simulink model "multi_rotor_sim"  (R2023b)
settings: Solver=ode4  StartTime=0.0  StopTime=inf  FixedStep=ST  RelTol=1e-3
values from neighbouring files (symbols this model uses):
  a0 = 0    [parameters.m]
  ASLOPE = 5.9    [parameters.m]
  Ax = 0.023    [parameters.m]
  Ay = 0.023    [parameters.m]
  Az = 0.106    [parameters.m]
  BLADES = 2    [parameters.m]
  BLCG = 0    [parameters.m]
  BLCP = 0    [parameters.m]
  BLH1 = b*sind(30)    [parameters.m]
  BLH2 = b    (= 0.275)    [parameters.m]
  BLH3 = b*sind(30)    [parameters.m]
  BLH4 = -b*sind(30)    [parameters.m]
  BLH5 = -b    (= -0.275)    [parameters.m]
  BLH6 = -b*sind(30)    [parameters.m]
  chi1 = 1    [parameters.m]
  chi2 = -1    [parameters.m]
  chi3 = 1    [parameters.m]
  chi4 = -1    [parameters.m]
  chi5 = 1    [parameters.m]
  chi6 = -1    [parameters.m]
  CHORD = 17.55e-3    (= 0.01755)    [parameters.m]
  CHORD75 = 21e-3    (= 0.021)    [parameters.m]
  dyn_viscosity = 17.89e-6    (= 1.789e-05)    [parameters.m]
  g0 = 9.80665    [parameters.m]
  href = 0    [parameters.m]
  k_ind = 1.35    [parameters.m]
  k_Omega = 14.92    [parameters.m]
  latref = 44.200626    [parameters.m]
  lonref = 12.063822    [parameters.m]
  m = 2.15    [parameters.m]
  MC_ATT_PITCH = 45*pi/180    (= 0.785398163397)    [parameters.m]
  MC_ATT_ROLL = 45*pi/180    (= 0.785398163397)    [parameters.m]
  MC_PITCH_P = 2    [parameters.m]
  MC_PITCHRATE_D = 0    [parameters.m]
  MC_PITCHRATE_I = 0.05    [parameters.m]
  MC_PITCHRATE_P = 0.09*3    (= 0.27)    [parameters.m]
  MC_RATE_PITCH = 500*pi/180    (= 8.72664625997)    [parameters.m]
  MC_RATE_ROLL = 500*pi/180    (= 8.72664625997)    [parameters.m]
  MC_RATE_YAW = 300*pi/180    (= 5.23598775598)    [parameters.m]
  MC_ROLL_P = 2    [parameters.m]
  MC_ROLLRATE_D = 0    [parameters.m]
  MC_ROLLRATE_I = 0.05    [parameters.m]
  MC_ROLLRATE_P = 0.09*3    (= 0.27)    [parameters.m]
  MC_VEL_FWD = 15    [parameters.m]
  MC_VEL_FWD_OPT = 0.5    [parameters.m]
  MC_VEL_LAT = 15    [parameters.m]
  MC_VEL_LAT_OPT = 0.5    [parameters.m]
  MC_VEL_VERT = 15    [parameters.m]
  MC_YAW_P = 0.55    [parameters.m]
  MC_YAWRATE_D = 0.05    [parameters.m]
  MC_YAWRATE_I = 0.02    [parameters.m]
  MC_YAWRATE_P = 0.15*3    (= 0.45)    [parameters.m]
  MPC_XY_VEL_D_ACC = 0.6    [parameters.m]
  MPC_XY_VEL_I_ACC = 0.8    [parameters.m]
  MPC_XY_VEL_P_ACC = 1.7    [parameters.m]
  MPC_Z_VEL_D_ACC = 0    [parameters.m]
  MPC_Z_VEL_I_ACC = 2    [parameters.m]
  MPC_Z_VEL_P_ACC = 4    [parameters.m]
  n = 0.6359    [parameters.m]
  p00 = 7.145e-2    (= 0.07145)    [parameters.m]
  p01 = 0.4377    [parameters.m]
  p02 = -10.13    [parameters.m]
  p10 = 1.259e-3    (= 0.001259)    [parameters.m]
  p11 = 1.284e-3    (= 0.001284)    [parameters.m]
  p20 = -7.513e-7    (= -7.513e-07)    [parameters.m]
  PWM_hover = (PWM_idle+PWM_max)/2    (= 1550)    [parameters.m]
  PWM_idle = 1100    [parameters.m]
  PWM_max = 2000    [parameters.m]
  ROTOR = 4*0.0254    (= 0.1016)    [parameters.m]
  ST = 0.01    [parameters.m]
  STACG = 0    [parameters.m]
  STACP = 0    [parameters.m]
  STAH1 = -b*cosd(30)    [parameters.m]
  STAH2 = 0    [parameters.m]
  STAH3 = b*cosd(30)    [parameters.m]
  STAH4 = b*cosd(30)    [parameters.m]
  STAH5 = 0    [parameters.m]
  STAH6 = -b*cosd(30)    [parameters.m]
  TERMINAL_SPEED = 0.5    [parameters.m]
  Theta0 = 45*pi/180    (= 0.785398163397)    [parameters.m]
  THETT = -38.0973*pi/180    (= -0.66492332112)    [parameters.m]
  wind_rate = [ 0 0 0 ]'    [parameters.m]
  wind_velocity_e = [ 0 0 0 ]'    [parameters.m]
  WLCG = -0.02    [parameters.m]
  WLCP = -0.08    [parameters.m]
  WLH1 = 32e-3    (= 0.032)    [parameters.m]
  WLH2 = 32e-3    (= 0.032)    [parameters.m]
  WLH3 = 32e-3    (= 0.032)    [parameters.m]
  WLH4 = 32e-3    (= 0.032)    [parameters.m]
  WLH5 = 32e-3    (= 0.032)    [parameters.m]
  WLH6 = 32e-3    (= 0.032)    [parameters.m]
undefined symbols (not defined in the file or in its folder): Earth, WGS84, X, Y, Z
libraries: sm_lib x258, slpidlib x36, nesl_utility x15, sharedtransform x13, aerolibutil x4, aerolibanimutils x3, sharedutil x2, sim3dlib x1, uavsim3dlib x1, shared6dof x1, aerolibtransform2 x1, aerolibatmos2 x1
(part 10 of 11)

== system multi_rotor_sim/3D_visualization/SIMECHANICS 3D SCENE/SimMechanics/MotorD/DCBL_Assembly_CounterClockwise_4_Top_1_RIGID/Assem4DCBL_Assembly_CounterClockwise_4_Top_1_RIGID ==
  Mieng_chan_canh_quat_1_RIGID : Subsystem
  ReferenceFrame : sm_lib/Frames and Transforms/Reference Frame
  Tang_tren_DCBL_1_RIGID : Subsystem
  Transform : sm_lib/Frames and Transforms/Rigid Transform  TranslationMethod=None  TranslationStandardOffset=0  TranslationStandardOffsetUnits=m  TranslationStandardAxis=+Z  TranslationCartesianOffset=[0 0 0]  TranslationCartesianOffsetUnits=m  TranslationROffset=0  TranslationROffsetUnits=m  TranslationZOffset=0  TranslationZOffsetUnits=m  TranslationThetaOffset=0  TranslationThetaOffsetUnits=deg  RotationMethod=None  RotationAngleUnits=deg  RotationStandardAxis=+Z  RotationAngle=0  RotationArbitraryAxis=[0 0 1]  FollAlignAxisA=+X  BaseAlignAxisA=+Y  FollAlignAxisB=+Y  BaseAlignAxisB=+Z  RotationSequenceAxes=FollowerAxes  RotationSequence=XYX  RotationSequenceAngles=[0 0 0]  RotationSequenceAnglesUnits=deg  RotationMatrix=[1 0 0; 0 1 0; 0 0 1]  Quaternion=[1 0 0 0]
  Transform1 : sm_lib/Frames and Transforms/Rigid Transform  TranslationMethod=Cartesian  TranslationStandardOffset=0  TranslationStandardOffsetUnits=mm  TranslationStandardAxis=+Z  TranslationCartesianOffset=[0 12.200000000000017 0]  TranslationCartesianOffsetUnits=mm  TranslationROffset=0  TranslationROffsetUnits=m  TranslationZOffset=0  TranslationZOffsetUnits=m  TranslationThetaOffset=0  TranslationThetaOffsetUnits=deg  RotationMethod=ArbitraryAxis  RotationAngleUnits=rad  RotationStandardAxis=+Z  RotationAngle=3.1415926535897931  RotationArbitraryAxis=[0 1 0]  FollAlignAxisA=+X  BaseAlignAxisA=+Y  FollAlignAxisB=+Y  BaseAlignAxisB=+Z  RotationSequenceAxes=FollowerAxes  RotationSequence=XYX  RotationSequenceAngles=[0 0 0]  RotationSequenceAnglesUnits=deg  RotationMatrix=[1 0 0; 0 1 0; 0 0 1]  Quaternion=[1 0 0 0]
  Transform2 : sm_lib/Frames and Transforms/Rigid Transform  TranslationMethod=Cartesian  TranslationStandardOffset=0  TranslationStandardOffsetUnits=mm  TranslationStandardAxis=+Z  TranslationCartesianOffset=[5.0000000000000044 5.5000000000000053 3.8000000000000118]  TranslationCartesianOffsetUnits=mm  TranslationROffset=0  TranslationROffsetUnits=m  TranslationZOffset=0  TranslationZOffsetUnits=m  TranslationThetaOffset=0  TranslationThetaOffsetUnits=deg  RotationMethod=ArbitraryAxis  RotationAngleUnits=rad  RotationStandardAxis=+Z  RotationAngle=3.1415926535897931  RotationArbitraryAxis=[0 1 0]  FollAlignAxisA=+X  BaseAlignAxisA=+Y  FollAlignAxisB=+Y  BaseAlignAxisB=+Z  RotationSequenceAxes=FollowerAxes  RotationSequence=XYX  RotationSequenceAngles=[0 0 0]  RotationSequenceAnglesUnits=deg  RotationMatrix=[1 0 0; 0 1 0; 0 0 1]  Quaternion=[1 0 0 0]
  Transform3 : sm_lib/Frames and Transforms/Rigid Transform  TranslationMethod=Cartesian  TranslationStandardOffset=0  TranslationStandardOffsetUnits=mm  TranslationStandardAxis=+Z  TranslationCartesianOffset=[0 16.899999999999999 0]  TranslationCartesianOffsetUnits=mm  TranslationROffset=0  TranslationROffsetUnits=m  TranslationZOffset=0  TranslationZOffsetUnits=m  TranslationThetaOffset=0  TranslationThetaOffsetUnits=deg  RotationMethod=ArbitraryAxis  RotationAngleUnits=rad  RotationStandardAxis=+Z  RotationAngle=2.0943951023931953  RotationArbitraryAxis=[-0.57735026918962584 0.57735026918962584 0.57735026918962584]  FollAlignAxisA=+X  BaseAlignAxisA=+Y  FollAlignAxisB=+Y  BaseAlignAxisB=+Z  RotationSequenceAxes=FollowerAxes  RotationSequence=XYX  RotationSequenceAngles=[0 0 0]  RotationSequenceAnglesUnits=deg  RotationMatrix=[1 0 0; 0 1 0; 0 0 1]  Quaternion=[1 0 0 0]
  Transform4 : sm_lib/Frames and Transforms/Rigid Transform  TranslationMethod=Cartesian  TranslationStandardOffset=0  TranslationStandardOffsetUnits=mm  TranslationStandardAxis=+Z  TranslationCartesianOffset=[0 30.500000000000014 0]  TranslationCartesianOffsetUnits=mm  TranslationROffset=0  TranslationROffsetUnits=m  TranslationZOffset=0  TranslationZOffsetUnits=m  TranslationThetaOffset=0  TranslationThetaOffsetUnits=deg  RotationMethod=ArbitraryAxis  RotationAngleUnits=rad  RotationStandardAxis=+Z  RotationAngle=2.994911156014171  RotationArbitraryAxis=[0 1 0]  FollAlignAxisA=+X  BaseAlignAxisA=+Y  FollAlignAxisB=+Y  BaseAlignAxisB=+Z  RotationSequenceAxes=FollowerAxes  RotationSequence=XYX  RotationSequenceAngles=[0 0 0]  RotationSequenceAnglesUnits=deg  RotationMatrix=[1 0 0; 0 1 0; 0 0 1]  Quaternion=[1 0 0 0]
  hex_nut_style_1_gradeab_iso_1_RIGID : Subsystem
  x10x4_7_counterclockwise_propeller_1_RIGID : Subsystem
  F : PMIOPort  Side=Left
  connections:
  Tang_tren_DCBL_1_RIGID/LConn1 -- Transform/RConn1
  Mieng_chan_canh_quat_1_RIGID/LConn1 -- Transform1/RConn1
  Transform2/RConn1 -- x10x4_7_counterclockwise_propeller_1_RIGID/LConn1
  Transform3/RConn1 -- hex_nut_style_1_gradeab_iso_1_RIGID/LConn1
  Transform/LConn1 -- Transform1/LConn1 -- Transform4/RConn1 -- ReferenceFrame/RConn1 -- Transform2/LConn1 -- Transform3/LConn1
  Transform4/LConn1 -- F/RConn1

== system multi_rotor_sim/3D_visualization/SIMECHANICS 3D SCENE/SimMechanics/Assembly_Quadrotor_NProp_1_RIGID/Assembly_Quadrotor_NoProp_1_RIGID/DCBL_Assembly_Clockwise_1_Bottom_1_RIGID/De_DCBL_1_RIGID ==
  ReferenceFrame : sm_lib/Frames and Transforms/Reference Frame
  Solid : sm_lib/Body Elements/File Solid  ExtGeomFileName=De_DCBL_Default_sldprt.STL  UnitType=Custom  ExtGeomFileUnits=mm  StepReaderType=HEX  ExportConvexHullGeometry=off  InertiaType=Custom  Mass=0.0094405067370886605  MassUnits=kg  CenterOfMass=[0 8.551755407943574 0]  CenterOfMassUnits=mm  MomentsOfInertia=[0.9581719720589793 0.57744869492610285 0.95817197205897908]  MomentsOfInertiaUnits=kg*mm^2  ProductsOfInertia=[0 -0.0012524646336928653 0]  ProductsOfInertiaUnits=kg*mm^2  BasedOnType=Density  Density=1000  DensityUnits=kg/(m^3)  DoExposeReferenceFrame=on  SerializedFrames=<Frames/>  GraphicType=FromGeometry  MarkerShape=Sphere  MarkerSize=10  MarkerSizeUnits=m  GraphicVisPropType=SimpleVisualProperties  GraphicDiffuseColor=[0.2 0.2 0.2]  GraphicSpecularColor=[0.5 0.5 0.5 1.0]  GraphicAmbientColor=[0.15 0.15 0.15 1.0]  GraphicEmissiveColor=[0.0 0.0 0.0 1.0]  GraphicShininess=75  GraphicOpacity=1
  F : PMIOPort  Side=Left
  connections:
  Solid/RConn1 -- ReferenceFrame/RConn1 -- F/RConn1

== system multi_rotor_sim/3D_visualization/SIMECHANICS 3D SCENE/SimMechanics/Assembly_Quadrotor_NProp_1_RIGID/Assembly_Quadrotor_NoProp_1_RIGID/DCBL_Assembly_Clockwise_3_Bottom_1_RIGID/De_DCBL_1_RIGID ==
  ReferenceFrame : sm_lib/Frames and Transforms/Reference Frame
  Solid : sm_lib/Body Elements/File Solid  ExtGeomFileName=De_DCBL_Default_sldprt.STL  UnitType=Custom  ExtGeomFileUnits=mm  StepReaderType=HEX  ExportConvexHullGeometry=off  InertiaType=Custom  Mass=0.0094405067370886605  MassUnits=kg  CenterOfMass=[0 8.551755407943574 0]  CenterOfMassUnits=mm  MomentsOfInertia=[0.9581719720589793 0.57744869492610285 0.95817197205897908]  MomentsOfInertiaUnits=kg*mm^2  ProductsOfInertia=[0 -0.0012524646336928653 0]  ProductsOfInertiaUnits=kg*mm^2  BasedOnType=Density  Density=1000  DensityUnits=kg/(m^3)  DoExposeReferenceFrame=on  SerializedFrames=<Frames/>  GraphicType=FromGeometry  MarkerShape=Sphere  MarkerSize=10  MarkerSizeUnits=m  GraphicVisPropType=SimpleVisualProperties  GraphicDiffuseColor=[0.2 0.2 0.2]  GraphicSpecularColor=[0.5 0.5 0.5 1.0]  GraphicAmbientColor=[0.15 0.15 0.15 1.0]  GraphicEmissiveColor=[0.0 0.0 0.0 1.0]  GraphicShininess=75  GraphicOpacity=1
  F : PMIOPort  Side=Left
  connections:
  Solid/RConn1 -- ReferenceFrame/RConn1 -- F/RConn1

== system multi_rotor_sim/3D_visualization/SIMECHANICS 3D SCENE/SimMechanics/Assembly_Quadrotor_NProp_1_RIGID/Assembly_Quadrotor_NoProp_1_RIGID/DCBL_Assembly_CounterClockwise_2_Bottom_1_RIGID/De_DCBL_1_RIGID ==
  ReferenceFrame : sm_lib/Frames and Transforms/Reference Frame
  Solid : sm_lib/Body Elements/File Solid  ExtGeomFileName=De_DCBL_Default_sldprt.STL  UnitType=Custom  ExtGeomFileUnits=mm  StepReaderType=HEX  ExportConvexHullGeometry=off  InertiaType=Custom  Mass=0.0094405067370886605  MassUnits=kg  CenterOfMass=[0 8.551755407943574 0]  CenterOfMassUnits=mm  MomentsOfInertia=[0.9581719720589793 0.57744869492610285 0.95817197205897908]  MomentsOfInertiaUnits=kg*mm^2  ProductsOfInertia=[0 -0.0012524646336928653 0]  ProductsOfInertiaUnits=kg*mm^2  BasedOnType=Density  Density=1000  DensityUnits=kg/(m^3)  DoExposeReferenceFrame=on  SerializedFrames=<Frames/>  GraphicType=FromGeometry  MarkerShape=Sphere  MarkerSize=10  MarkerSizeUnits=m  GraphicVisPropType=SimpleVisualProperties  GraphicDiffuseColor=[0.2 0.2 0.2]  GraphicSpecularColor=[0.5 0.5 0.5 1.0]  GraphicAmbientColor=[0.15 0.15 0.15 1.0]  GraphicEmissiveColor=[0.0 0.0 0.0 1.0]  GraphicShininess=75  GraphicOpacity=1
  F : PMIOPort  Side=Left
  connections:
  Solid/RConn1 -- ReferenceFrame/RConn1 -- F/RConn1

== system multi_rotor_sim/3D_visualization/SIMECHANICS 3D SCENE/SimMechanics/Assembly_Quadrotor_NProp_1_RIGID/Assembly_Quadrotor_NoProp_1_RIGID/DCBL_Assembly_CounterClockwise_4_Bottom_1_RIGID/De_DCBL_1_RIGID ==
  ReferenceFrame : sm_lib/Frames and Transforms/Reference Frame
  Solid : sm_lib/Body Elements/File Solid  ExtGeomFileName=De_DCBL_Default_sldprt.STL  UnitType=Custom  ExtGeomFileUnits=mm  StepReaderType=HEX  ExportConvexHullGeometry=off  InertiaType=Custom  Mass=0.0094405067370886605  MassUnits=kg  CenterOfMass=[0 8.551755407943574 0]  CenterOfMassUnits=mm  MomentsOfInertia=[0.9581719720589793 0.57744869492610285 0.95817197205897908]  MomentsOfInertiaUnits=kg*mm^2  ProductsOfInertia=[0 -0.0012524646336928653 0]  ProductsOfInertiaUnits=kg*mm^2  BasedOnType=Density  Density=1000  DensityUnits=kg/(m^3)  DoExposeReferenceFrame=on  SerializedFrames=<Frames/>  GraphicType=FromGeometry  MarkerShape=Sphere  MarkerSize=10  MarkerSizeUnits=m  GraphicVisPropType=SimpleVisualProperties  GraphicDiffuseColor=[0.2 0.2 0.2]  GraphicSpecularColor=[0.5 0.5 0.5 1.0]  GraphicAmbientColor=[0.15 0.15 0.15 1.0]  GraphicEmissiveColor=[0.0 0.0 0.0 1.0]  GraphicShininess=75  GraphicOpacity=1
  F : PMIOPort  Side=Left
  connections:
  Solid/RConn1 -- ReferenceFrame/RConn1 -- F/RConn1

== system multi_rotor_sim/3D_visualization/SIMECHANICS 3D SCENE/SimMechanics/MotorA/DCBL_Assembly_Clockwise_1_Top_1_RIGID/Assem1DCBL_Assembly_Clockwise_1_Top_1_RIGID/Mieng_chan_canh_quat_1_RIGID ==
  ReferenceFrame : sm_lib/Frames and Transforms/Reference Frame
  Solid : sm_lib/Body Elements/File Solid  ExtGeomFileName=Mieng_chan_canh_quat_Default_sldprt.STL  UnitType=Custom  ExtGeomFileUnits=mm  StepReaderType=HEX  ExportConvexHullGeometry=off  InertiaType=Custom  Mass=0.00066710164886432991  MassUnits=kg  CenterOfMass=[0 0.34100350204192958 0]  CenterOfMassUnits=mm  MomentsOfInertia=[0.0086037825507957657 0.016809111968954363 0.0086037825507957692]  MomentsOfInertiaUnits=kg*mm^2  ProductsOfInertia=[0 0 0]  ProductsOfInertiaUnits=kg*mm^2  BasedOnType=Density  Density=1000  DensityUnits=kg/(m^3)  DoExposeReferenceFrame=on  SerializedFrames=<Frames/>  GraphicType=FromGeometry  MarkerShape=Sphere  MarkerSize=10  MarkerSizeUnits=m  GraphicVisPropType=SimpleVisualProperties  GraphicDiffuseColor=[0.1 0.1 0.1]  GraphicSpecularColor=[0.5 0.5 0.5 1.0]  GraphicAmbientColor=[0.15 0.15 0.15 1.0]  GraphicEmissiveColor=[0.0 0.0 0.0 1.0]  GraphicShininess=75  GraphicOpacity=1
  F : PMIOPort  Side=Left
  connections:
  Solid/RConn1 -- ReferenceFrame/RConn1 -- F/RConn1

== system multi_rotor_sim/3D_visualization/SIMECHANICS 3D SCENE/SimMechanics/MotorA/DCBL_Assembly_Clockwise_1_Top_1_RIGID/Assem1DCBL_Assembly_Clockwise_1_Top_1_RIGID/Tang_tren_DCBL_1_RIGID ==
  ReferenceFrame : sm_lib/Frames and Transforms/Reference Frame
  Solid : sm_lib/Body Elements/File Solid  ExtGeomFileName=Tang_tren_DCBL_Default_sldprt.STL  UnitType=Custom  ExtGeomFileUnits=mm  StepReaderType=HEX  ExportConvexHullGeometry=off  InertiaType=Custom  Mass=0.0096533797201190392  MassUnits=kg  CenterOfMass=[0 -3.2502099324489322 0]  CenterOfMassUnits=mm  MomentsOfInertia=[1.2743807926810715 0.81038583319969226 1.2743807926810709]  MomentsOfInertiaUnits=kg*mm^2  ProductsOfInertia=[0 0 0]  ProductsOfInertiaUnits=kg*mm^2  BasedOnType=Density  Density=1000  DensityUnits=kg/(m^3)  DoExposeReferenceFrame=on  SerializedFrames=<Frames/>  GraphicType=FromGeometry  MarkerShape=Sphere  MarkerSize=10  MarkerSizeUnits=m  GraphicVisPropType=SimpleVisualProperties  GraphicDiffuseColor=[0.1 0.1 0.1]  GraphicSpecularColor=[0.5 0.5 0.5 1.0]  GraphicAmbientColor=[0.15 0.15 0.15 1.0]  GraphicEmissiveColor=[0.0 0.0 0.0 1.0]  GraphicShininess=75  GraphicOpacity=1
  F : PMIOPort  Side=Left
  connections:
  Solid/RConn1 -- ReferenceFrame/RConn1 -- F/RConn1

== system multi_rotor_sim/3D_visualization/SIMECHANICS 3D SCENE/SimMechanics/MotorA/DCBL_Assembly_Clockwise_1_Top_1_RIGID/Assem1DCBL_Assembly_Clockwise_1_Top_1_RIGID/hex_nut_style_1_gradeab_iso_1_RIGID ==
  ReferenceFrame : sm_lib/Frames and Transforms/Reference Frame
  Solid : sm_lib/Body Elements/File Solid  ExtGeomFileName=hex nut style 1 gradeab_iso_Hexagon Nut ISO - 4032 - M4 - D - N_sldprt.STL  UnitType=Custom  ExtGeomFileUnits=mm  StepReaderType=HEX  ExportConvexHullGeometry=off  InertiaType=Custom  Mass=0.00010662444846940384  MassUnits=kg  CenterOfMass=[0 1.3702747535691162e-06 -1.5985959803450969]  CenterOfMassUnits=mm  MomentsOfInertia=[0.00052487586358693401 0.00052487294180577238 0.00087302244809774987]  MomentsOfInertiaUnits=kg*mm^2  ProductsOfInertia=[0 0 0]  ProductsOfInertiaUnits=kg*mm^2  BasedOnType=Density  Density=1000  DensityUnits=kg/(m^3)  DoExposeReferenceFrame=on  SerializedFrames=<Frames/>  GraphicType=FromGeometry  MarkerShape=Sphere  MarkerSize=10  MarkerSizeUnits=m  GraphicVisPropType=SimpleVisualProperties  GraphicDiffuseColor=[0.77647058823529413 0.75686274509803919 0.73725490196078436]  GraphicSpecularColor=[0.5 0.5 0.5 1.0]  GraphicAmbientColor=[0.15 0.15 0.15 1.0]  GraphicEmissiveColor=[0.0 0.0 0.0 1.0]  GraphicShininess=75  GraphicOpacity=1
  F : PMIOPort  Side=Left
  connections:
  Solid/RConn1 -- ReferenceFrame/RConn1 -- F/RConn1

== system multi_rotor_sim/3D_visualization/SIMECHANICS 3D SCENE/SimMechanics/MotorA/DCBL_Assembly_Clockwise_1_Top_1_RIGID/Assem1DCBL_Assembly_Clockwise_1_Top_1_RIGID/x10x4_7_clockwise_propeller_1_RIGID ==
  ReferenceFrame : sm_lib/Frames and Transforms/Reference Frame
  Solid : sm_lib/Body Elements/File Solid  ExtGeomFileName=10x4.7-clockwise-propeller_Default_sldprt.STL  UnitType=Custom  ExtGeomFileUnits=mm  StepReaderType=HEX  ExportConvexHullGeometry=off  InertiaType=Custom  Mass=0.0085886554018527825  MassUnits=kg  CenterOfMass=[5.0000101361481475 5.1432840109255382 3.799999228152465]  CenterOfMassUnits=mm  MomentsOfInertia=[37.986675876119939 39.040615812058284 1.1185316341050053]  MomentsOfInertiaUnits=kg*mm^2  ProductsOfInertia=[-7.8946012766185134e-07 -5.513228057178063 2.3221541821947674e-07]  ProductsOfInertiaUnits=kg*mm^2  BasedOnType=Density  Density=1000  DensityUnits=kg/(m^3)  DoExposeReferenceFrame=on  SerializedFrames=<Frames/>  GraphicType=FromGeometry  MarkerShape=Sphere  MarkerSize=10  MarkerSizeUnits=m  GraphicVisPropType=SimpleVisualProperties  GraphicDiffuseColor=[0.75294117647058822 0.75294117647058822 0.75294117647058822]  GraphicSpecularColor=[0.5 0.5 0.5 1.0]  GraphicAmbientColor=[0.15 0.15 0.15 1.0]  GraphicEmissiveColor=[0.0 0.0 0.0 1.0]  GraphicShininess=75  GraphicOpacity=1
  F : PMIOPort  Side=Left
  connections:
  Solid/RConn1 -- ReferenceFrame/RConn1 -- F/RConn1

== system multi_rotor_sim/3D_visualization/SIMECHANICS 3D SCENE/SimMechanics/MotorB/DCBL_Assembly_CounterClockwise_2_Top_1_RIGID/Assem2DCBL_Assembly_CounterClockwise_2_Top_1_RIGID/Mieng_chan_canh_quat_1_RIGID ==
  ReferenceFrame : sm_lib/Frames and Transforms/Reference Frame
  Solid : sm_lib/Body Elements/File Solid  ExtGeomFileName=Mieng_chan_canh_quat_Default_sldprt.STL  UnitType=Custom  ExtGeomFileUnits=mm  StepReaderType=HEX  ExportConvexHullGeometry=off  InertiaType=Custom  Mass=0.00066710164886432991  MassUnits=kg  CenterOfMass=[0 0.34100350204192958 0]  CenterOfMassUnits=mm  MomentsOfInertia=[0.0086037825507957657 0.016809111968954363 0.0086037825507957692]  MomentsOfInertiaUnits=kg*mm^2  ProductsOfInertia=[0 0 0]  ProductsOfInertiaUnits=kg*mm^2  BasedOnType=Density  Density=1000  DensityUnits=kg/(m^3)  DoExposeReferenceFrame=on  SerializedFrames=<Frames/>  GraphicType=FromGeometry  MarkerShape=Sphere  MarkerSize=10  MarkerSizeUnits=m  GraphicVisPropType=SimpleVisualProperties  GraphicDiffuseColor=[0.1 0.1 0.1]  GraphicSpecularColor=[0.5 0.5 0.5 1.0]  GraphicAmbientColor=[0.15 0.15 0.15 1.0]  GraphicEmissiveColor=[0.0 0.0 0.0 1.0]  GraphicShininess=75  GraphicOpacity=1
  F : PMIOPort  Side=Left
  connections:
  Solid/RConn1 -- ReferenceFrame/RConn1 -- F/RConn1

== system multi_rotor_sim/3D_visualization/SIMECHANICS 3D SCENE/SimMechanics/MotorB/DCBL_Assembly_CounterClockwise_2_Top_1_RIGID/Assem2DCBL_Assembly_CounterClockwise_2_Top_1_RIGID/Tang_tren_DCBL_1_RIGID ==
  ReferenceFrame : sm_lib/Frames and Transforms/Reference Frame
  Solid : sm_lib/Body Elements/File Solid  ExtGeomFileName=Tang_tren_DCBL_Default_sldprt.STL  UnitType=Custom  ExtGeomFileUnits=mm  StepReaderType=HEX  ExportConvexHullGeometry=off  InertiaType=Custom  Mass=0.0096533797201190392  MassUnits=kg  CenterOfMass=[0 -3.2502099324489322 0]  CenterOfMassUnits=mm  MomentsOfInertia=[1.2743807926810715 0.81038583319969226 1.2743807926810709]  MomentsOfInertiaUnits=kg*mm^2  ProductsOfInertia=[0 0 0]  ProductsOfInertiaUnits=kg*mm^2  BasedOnType=Density  Density=1000  DensityUnits=kg/(m^3)  DoExposeReferenceFrame=on  SerializedFrames=<Frames/>  GraphicType=FromGeometry  MarkerShape=Sphere  MarkerSize=10  MarkerSizeUnits=m  GraphicVisPropType=SimpleVisualProperties  GraphicDiffuseColor=[0.1 0.1 0.1]  GraphicSpecularColor=[0.5 0.5 0.5 1.0]  GraphicAmbientColor=[0.15 0.15 0.15 1.0]  GraphicEmissiveColor=[0.0 0.0 0.0 1.0]  GraphicShininess=75  GraphicOpacity=1
  F : PMIOPort  Side=Left
  connections:
  Solid/RConn1 -- ReferenceFrame/RConn1 -- F/RConn1

== system multi_rotor_sim/3D_visualization/SIMECHANICS 3D SCENE/SimMechanics/MotorB/DCBL_Assembly_CounterClockwise_2_Top_1_RIGID/Assem2DCBL_Assembly_CounterClockwise_2_Top_1_RIGID/hex_nut_style_1_gradeab_iso_1_RIGID ==
  ReferenceFrame : sm_lib/Frames and Transforms/Reference Frame
  Solid : sm_lib/Body Elements/File Solid  ExtGeomFileName=hex nut style 1 gradeab_iso_Hexagon Nut ISO - 4032 - M4 - D - N_sldprt.STL  UnitType=Custom  ExtGeomFileUnits=mm  StepReaderType=HEX  ExportConvexHullGeometry=off  InertiaType=Custom  Mass=0.00010662444846940384  MassUnits=kg  CenterOfMass=[0 1.3702747535691162e-06 -1.5985959803450969]  CenterOfMassUnits=mm  MomentsOfInertia=[0.00052487586358693401 0.00052487294180577238 0.00087302244809774987]  MomentsOfInertiaUnits=kg*mm^2  ProductsOfInertia=[0 0 0]  ProductsOfInertiaUnits=kg*mm^2  BasedOnType=Density  Density=1000  DensityUnits=kg/(m^3)  DoExposeReferenceFrame=on  SerializedFrames=<Frames/>  GraphicType=FromGeometry  MarkerShape=Sphere  MarkerSize=10  MarkerSizeUnits=m  GraphicVisPropType=SimpleVisualProperties  GraphicDiffuseColor=[0.77647058823529413 0.75686274509803919 0.73725490196078436]  GraphicSpecularColor=[0.5 0.5 0.5 1.0]  GraphicAmbientColor=[0.15 0.15 0.15 1.0]  GraphicEmissiveColor=[0.0 0.0 0.0 1.0]  GraphicShininess=75  GraphicOpacity=1
  F : PMIOPort  Side=Left
  connections:
  Solid/RConn1 -- ReferenceFrame/RConn1 -- F/RConn1

== system multi_rotor_sim/3D_visualization/SIMECHANICS 3D SCENE/SimMechanics/MotorB/DCBL_Assembly_CounterClockwise_2_Top_1_RIGID/Assem2DCBL_Assembly_CounterClockwise_2_Top_1_RIGID/x10x4_7_counterclockwise_propeller_1_RIGID ==
  ReferenceFrame : sm_lib/Frames and Transforms/Reference Frame
  Solid : sm_lib/Body Elements/File Solid  ExtGeomFileName=10x4.7-counterclockwise-propeller_Default_sldprt.STL  UnitType=Custom  ExtGeomFileUnits=mm  StepReaderType=HEX  ExportConvexHullGeometry=off  InertiaType=Custom  Mass=0.0086221636611543556  MassUnits=kg  CenterOfMass=[5.0000063702530122 5.136767030722547 3.7999863031218535]  CenterOfMassUnits=mm  MomentsOfInertia=[38.086408780943664 39.145966882895458 1.124519086575168]  MomentsOfInertiaUnits=kg*mm^2  ProductsOfInertia=[-1.7703894482553841e-07 5.5344154529569156 1.457353668708178e-07]  ProductsOfInertiaUnits=kg*mm^2  BasedOnType=Density  Density=1000  DensityUnits=kg/(m^3)  DoExposeReferenceFrame=on  SerializedFrames=<Frames/>  GraphicType=FromGeometry  MarkerShape=Sphere  MarkerSize=10  MarkerSizeUnits=m  GraphicVisPropType=SimpleVisualProperties  GraphicDiffuseColor=[0.75294117647058822 0.75294117647058822 0.75294117647058822]  GraphicSpecularColor=[0.5 0.5 0.5 1.0]  GraphicAmbientColor=[0.15 0.15 0.15 1.0]  GraphicEmissiveColor=[0.0 0.0 0.0 1.0]  GraphicShininess=75  GraphicOpacity=1
  F : PMIOPort  Side=Left
  connections:
  Solid/RConn1 -- ReferenceFrame/RConn1 -- F/RConn1

== system multi_rotor_sim/3D_visualization/SIMECHANICS 3D SCENE/SimMechanics/MotorC/DCBL_Assembly_Clockwise_3_Top_1_RIGID/Assem3DCBL_Assembly_Clockwise_3_Top_1_RIGID/Mieng_chan_canh_quat_1_RIGID ==
  ReferenceFrame : sm_lib/Frames and Transforms/Reference Frame
  Solid : sm_lib/Body Elements/File Solid  ExtGeomFileName=Mieng_chan_canh_quat_Default_sldprt.STL  UnitType=Custom  ExtGeomFileUnits=mm  StepReaderType=HEX  ExportConvexHullGeometry=off  InertiaType=Custom  Mass=0.00066710164886432991  MassUnits=kg  CenterOfMass=[0 0.34100350204192958 0]  CenterOfMassUnits=mm  MomentsOfInertia=[0.0086037825507957657 0.016809111968954363 0.0086037825507957692]  MomentsOfInertiaUnits=kg*mm^2  ProductsOfInertia=[0 0 0]  ProductsOfInertiaUnits=kg*mm^2  BasedOnType=Density  Density=1000  DensityUnits=kg/(m^3)  DoExposeReferenceFrame=on  SerializedFrames=<Frames/>  GraphicType=FromGeometry  MarkerShape=Sphere  MarkerSize=10  MarkerSizeUnits=m  GraphicVisPropType=SimpleVisualProperties  GraphicDiffuseColor=[0.1 0.1 0.1]  GraphicSpecularColor=[0.5 0.5 0.5 1.0]  GraphicAmbientColor=[0.15 0.15 0.15 1.0]  GraphicEmissiveColor=[0.0 0.0 0.0 1.0]  GraphicShininess=75  GraphicOpacity=1
  F : PMIOPort  Side=Left
  connections:
  Solid/RConn1 -- ReferenceFrame/RConn1 -- F/RConn1

== system multi_rotor_sim/3D_visualization/SIMECHANICS 3D SCENE/SimMechanics/MotorC/DCBL_Assembly_Clockwise_3_Top_1_RIGID/Assem3DCBL_Assembly_Clockwise_3_Top_1_RIGID/Tang_tren_DCBL_1_RIGID ==
  ReferenceFrame : sm_lib/Frames and Transforms/Reference Frame
  Solid : sm_lib/Body Elements/File Solid  ExtGeomFileName=Tang_tren_DCBL_Default_sldprt.STL  UnitType=Custom  ExtGeomFileUnits=mm  StepReaderType=HEX  ExportConvexHullGeometry=off  InertiaType=Custom  Mass=0.0096533797201190392  MassUnits=kg  CenterOfMass=[0 -3.2502099324489322 0]  CenterOfMassUnits=mm  MomentsOfInertia=[1.2743807926810715 0.81038583319969226 1.2743807926810709]  MomentsOfInertiaUnits=kg*mm^2  ProductsOfInertia=[0 0 0]  ProductsOfInertiaUnits=kg*mm^2  BasedOnType=Density  Density=1000  DensityUnits=kg/(m^3)  DoExposeReferenceFrame=on  SerializedFrames=<Frames/>  GraphicType=FromGeometry  MarkerShape=Sphere  MarkerSize=10  MarkerSizeUnits=m  GraphicVisPropType=SimpleVisualProperties  GraphicDiffuseColor=[0.1 0.1 0.1]  GraphicSpecularColor=[0.5 0.5 0.5 1.0]  GraphicAmbientColor=[0.15 0.15 0.15 1.0]  GraphicEmissiveColor=[0.0 0.0 0.0 1.0]  GraphicShininess=75  GraphicOpacity=1
  F : PMIOPort  Side=Left
  connections:
  Solid/RConn1 -- ReferenceFrame/RConn1 -- F/RConn1

== system multi_rotor_sim/3D_visualization/SIMECHANICS 3D SCENE/SimMechanics/MotorC/DCBL_Assembly_Clockwise_3_Top_1_RIGID/Assem3DCBL_Assembly_Clockwise_3_Top_1_RIGID/hex_nut_style_1_gradeab_iso_1_RIGID ==
  ReferenceFrame : sm_lib/Frames and Transforms/Reference Frame
  Solid : sm_lib/Body Elements/File Solid  ExtGeomFileName=hex nut style 1 gradeab_iso_Hexagon Nut ISO - 4032 - M4 - D - N_sldprt.STL  UnitType=Custom  ExtGeomFileUnits=mm  StepReaderType=HEX  ExportConvexHullGeometry=off  InertiaType=Custom  Mass=0.00010662444846940384  MassUnits=kg  CenterOfMass=[0 1.3702747535691162e-06 -1.5985959803450969]  CenterOfMassUnits=mm  MomentsOfInertia=[0.00052487586358693401 0.00052487294180577238 0.00087302244809774987]  MomentsOfInertiaUnits=kg*mm^2  ProductsOfInertia=[0 0 0]  ProductsOfInertiaUnits=kg*mm^2  BasedOnType=Density  Density=1000  DensityUnits=kg/(m^3)  DoExposeReferenceFrame=on  SerializedFrames=<Frames/>  GraphicType=FromGeometry  MarkerShape=Sphere  MarkerSize=10  MarkerSizeUnits=m  GraphicVisPropType=SimpleVisualProperties  GraphicDiffuseColor=[0.77647058823529413 0.75686274509803919 0.73725490196078436]  GraphicSpecularColor=[0.5 0.5 0.5 1.0]  GraphicAmbientColor=[0.15 0.15 0.15 1.0]  GraphicEmissiveColor=[0.0 0.0 0.0 1.0]  GraphicShininess=75  GraphicOpacity=1
  F : PMIOPort  Side=Left
  connections:
  Solid/RConn1 -- ReferenceFrame/RConn1 -- F/RConn1

== system multi_rotor_sim/3D_visualization/SIMECHANICS 3D SCENE/SimMechanics/MotorC/DCBL_Assembly_Clockwise_3_Top_1_RIGID/Assem3DCBL_Assembly_Clockwise_3_Top_1_RIGID/x10x4_7_clockwise_propeller_1_RIGID ==
  ReferenceFrame : sm_lib/Frames and Transforms/Reference Frame
  Solid : sm_lib/Body Elements/File Solid  ExtGeomFileName=10x4.7-clockwise-propeller_Default_sldprt.STL  UnitType=Custom  ExtGeomFileUnits=mm  StepReaderType=HEX  ExportConvexHullGeometry=off  InertiaType=Custom  Mass=0.0085886554018527825  MassUnits=kg  CenterOfMass=[5.0000101361481475 5.1432840109255382 3.799999228152465]  CenterOfMassUnits=mm  MomentsOfInertia=[37.986675876119939 39.040615812058284 1.1185316341050053]  MomentsOfInertiaUnits=kg*mm^2  ProductsOfInertia=[-7.8946012766185134e-07 -5.513228057178063 2.3221541821947674e-07]  ProductsOfInertiaUnits=kg*mm^2  BasedOnType=Density  Density=1000  DensityUnits=kg/(m^3)  DoExposeReferenceFrame=on  SerializedFrames=<Frames/>  GraphicType=FromGeometry  MarkerShape=Sphere  MarkerSize=10  MarkerSizeUnits=m  GraphicVisPropType=SimpleVisualProperties  GraphicDiffuseColor=[0.75294117647058822 0.75294117647058822 0.75294117647058822]  GraphicSpecularColor=[0.5 0.5 0.5 1.0]  GraphicAmbientColor=[0.15 0.15 0.15 1.0]  GraphicEmissiveColor=[0.0 0.0 0.0 1.0]  GraphicShininess=75  GraphicOpacity=1
  F : PMIOPort  Side=Left
  connections:
  Solid/RConn1 -- ReferenceFrame/RConn1 -- F/RConn1

== system multi_rotor_sim/3D_visualization/SIMECHANICS 3D SCENE/SimMechanics/MotorD/DCBL_Assembly_CounterClockwise_4_Top_1_RIGID/Assem4DCBL_Assembly_CounterClockwise_4_Top_1_RIGID/Mieng_chan_canh_quat_1_RIGID ==
  ReferenceFrame : sm_lib/Frames and Transforms/Reference Frame
  Solid : sm_lib/Body Elements/File Solid  ExtGeomFileName=Mieng_chan_canh_quat_Default_sldprt.STL  UnitType=Custom  ExtGeomFileUnits=mm  StepReaderType=HEX  ExportConvexHullGeometry=off  InertiaType=Custom  Mass=0.00066710164886432991  MassUnits=kg  CenterOfMass=[0 0.34100350204192958 0]  CenterOfMassUnits=mm  MomentsOfInertia=[0.0086037825507957657 0.016809111968954363 0.0086037825507957692]  MomentsOfInertiaUnits=kg*mm^2  ProductsOfInertia=[0 0 0]  ProductsOfInertiaUnits=kg*mm^2  BasedOnType=Density  Density=1000  DensityUnits=kg/(m^3)  DoExposeReferenceFrame=on  SerializedFrames=<Frames/>  GraphicType=FromGeometry  MarkerShape=Sphere  MarkerSize=10  MarkerSizeUnits=m  GraphicVisPropType=SimpleVisualProperties  GraphicDiffuseColor=[0.1 0.1 0.1]  GraphicSpecularColor=[0.5 0.5 0.5 1.0]  GraphicAmbientColor=[0.15 0.15 0.15 1.0]  GraphicEmissiveColor=[0.0 0.0 0.0 1.0]  GraphicShininess=75  GraphicOpacity=1
  F : PMIOPort  Side=Left
  connections:
  Solid/RConn1 -- ReferenceFrame/RConn1 -- F/RConn1

== system multi_rotor_sim/3D_visualization/SIMECHANICS 3D SCENE/SimMechanics/MotorD/DCBL_Assembly_CounterClockwise_4_Top_1_RIGID/Assem4DCBL_Assembly_CounterClockwise_4_Top_1_RIGID/Tang_tren_DCBL_1_RIGID ==
  ReferenceFrame : sm_lib/Frames and Transforms/Reference Frame
  Solid : sm_lib/Body Elements/File Solid  ExtGeomFileName=Tang_tren_DCBL_Default_sldprt.STL  UnitType=Custom  ExtGeomFileUnits=mm  StepReaderType=HEX  ExportConvexHullGeometry=off  InertiaType=Custom  Mass=0.0096533797201190392  MassUnits=kg  CenterOfMass=[0 -3.2502099324489322 0]  CenterOfMassUnits=mm  MomentsOfInertia=[1.2743807926810715 0.81038583319969226 1.2743807926810709]  MomentsOfInertiaUnits=kg*mm^2  ProductsOfInertia=[0 0 0]  ProductsOfInertiaUnits=kg*mm^2  BasedOnType=Density  Density=1000  DensityUnits=kg/(m^3)  DoExposeReferenceFrame=on  SerializedFrames=<Frames/>  GraphicType=FromGeometry  MarkerShape=Sphere  MarkerSize=10  MarkerSizeUnits=m  GraphicVisPropType=SimpleVisualProperties  GraphicDiffuseColor=[0.1 0.1 0.1]  GraphicSpecularColor=[0.5 0.5 0.5 1.0]  GraphicAmbientColor=[0.15 0.15 0.15 1.0]  GraphicEmissiveColor=[0.0 0.0 0.0 1.0]  GraphicShininess=75  GraphicOpacity=1
  F : PMIOPort  Side=Left
  connections:
  Solid/RConn1 -- ReferenceFrame/RConn1 -- F/RConn1

== system multi_rotor_sim/3D_visualization/SIMECHANICS 3D SCENE/SimMechanics/MotorD/DCBL_Assembly_CounterClockwise_4_Top_1_RIGID/Assem4DCBL_Assembly_CounterClockwise_4_Top_1_RIGID/hex_nut_style_1_gradeab_iso_1_RIGID ==
  ReferenceFrame : sm_lib/Frames and Transforms/Reference Frame
  Solid : sm_lib/Body Elements/File Solid  ExtGeomFileName=hex nut style 1 gradeab_iso_Hexagon Nut ISO - 4032 - M4 - D - N_sldprt.STL  UnitType=Custom  ExtGeomFileUnits=mm  StepReaderType=HEX  ExportConvexHullGeometry=off  InertiaType=Custom  Mass=0.00010662444846940384  MassUnits=kg  CenterOfMass=[0 1.3702747535691162e-06 -1.5985959803450969]  CenterOfMassUnits=mm  MomentsOfInertia=[0.00052487586358693401 0.00052487294180577238 0.00087302244809774987]  MomentsOfInertiaUnits=kg*mm^2  ProductsOfInertia=[0 0 0]  ProductsOfInertiaUnits=kg*mm^2  BasedOnType=Density  Density=1000  DensityUnits=kg/(m^3)  DoExposeReferenceFrame=on  SerializedFrames=<Frames/>  GraphicType=FromGeometry  MarkerShape=Sphere  MarkerSize=10  MarkerSizeUnits=m  GraphicVisPropType=SimpleVisualProperties  GraphicDiffuseColor=[0.77647058823529413 0.75686274509803919 0.73725490196078436]  GraphicSpecularColor=[0.5 0.5 0.5 1.0]  GraphicAmbientColor=[0.15 0.15 0.15 1.0]  GraphicEmissiveColor=[0.0 0.0 0.0 1.0]  GraphicShininess=75  GraphicOpacity=1
  F : PMIOPort  Side=Left
  connections:
  Solid/RConn1 -- ReferenceFrame/RConn1 -- F/RConn1

== system multi_rotor_sim/3D_visualization/SIMECHANICS 3D SCENE/SimMechanics/MotorD/DCBL_Assembly_CounterClockwise_4_Top_1_RIGID/Assem4DCBL_Assembly_CounterClockwise_4_Top_1_RIGID/x10x4_7_counterclockwise_propeller_1_RIGID ==
  ReferenceFrame : sm_lib/Frames and Transforms/Reference Frame
  Solid : sm_lib/Body Elements/File Solid  ExtGeomFileName=10x4.7-counterclockwise-propeller_Default_sldprt.STL  UnitType=Custom  ExtGeomFileUnits=mm  StepReaderType=HEX  ExportConvexHullGeometry=off  InertiaType=Custom  Mass=0.0086221636611543556  MassUnits=kg  CenterOfMass=[5.0000063702530122 5.136767030722547 3.7999863031218535]  CenterOfMassUnits=mm  MomentsOfInertia=[38.086408780943664 39.145966882895458 1.124519086575168]  MomentsOfInertiaUnits=kg*mm^2  ProductsOfInertia=[-1.7703894482553841e-07 5.5344154529569156 1.457353668708178e-07]  ProductsOfInertiaUnits=kg*mm^2  BasedOnType=Density  Density=1000  DensityUnits=kg/(m^3)  DoExposeReferenceFrame=on  SerializedFrames=<Frames/>  GraphicType=FromGeometry  MarkerShape=Sphere  MarkerSize=10  MarkerSizeUnits=m  GraphicVisPropType=SimpleVisualProperties  GraphicDiffuseColor=[0.75294117647058822 0.75294117647058822 0.75294117647058822]  GraphicSpecularColor=[0.5 0.5 0.5 1.0]  GraphicAmbientColor=[0.15 0.15 0.15 1.0]  GraphicEmissiveColor=[0.0 0.0 0.0 1.0]  GraphicShininess=75  GraphicOpacity=1
  F : PMIOPort  Side=Left
  connections:
  Solid/RConn1 -- ReferenceFrame/RConn1 -- F/RConn1

== matlab function multi_rotor_sim/MULTIROTOR MODEL/ROTORS FORCE AND MOMENT/ROTOR2/MATLAB Function ==
  data: BLADES input; Mrotor output; ASLOPE input; CHORD input; CHORD75 input; ROTOR input; a0 input; Theta0 input; THETT input; dyn_viscosity input; k_ind input; STACG input; BLCG input; WLCG input; STAH input; BLH input; WLH input; chi input; rho input; TAS input; omega_TAS input; Frotor output; Q output; omega input; Omega input
function [Mrotor,Frotor,Q] = fcn(BLADES,ASLOPE,CHORD,CHORD75,ROTOR,a0,Theta0,THETT,dyn_viscosity,k_ind,STACG,BLCG,WLCG,STAH,BLH,WLH,chi,rho,TAS,omega_TAS,omega,Omega)

%% preliminary calculations
A = pi*ROTOR^2; % area of rotor disc 
sigma = BLADES*CHORD/(pi*ROTOR); % solidity of rotor 
lever_arm_H = [STACG-STAH BLH-BLCG WLCG-WLH]'; % vector from cg to rotor hub
TAS_H = [1 chi 1]'.*(TAS + cross(omega_TAS,lever_arm_H)); % wind speed at rotor
uH = TAS_H(1);
vH = TAS_H(2);
wH = TAS_H(3);
beta_w = atan2(vH,uH); % sideslip angle 
Mu = sqrt(uH^2+vH^2)/(Omega*ROTOR); % advance ratio
p = omega(1); % roll rate
q = omega(2); % pitch rate
pH = chi*p;
qH = q;

%% thrust calculation

lambda = fzero(@(x) x-wH/(Omega*ROTOR)+0.5*((0.5*BLADES*rho*ASLOPE*CHORD*ROTOR*(Omega*ROTOR)^2*(x/2+ ...
         +Theta0*(1/3+Mu^2/2)+THETT*(1/4+Mu^2/4)+Mu/4*(pH/Omega*cos(beta_w)+ ...
         +qH/Omega*sin(beta_w))))/(rho*A*(Omega*ROTOR)^2))/sqrt(Mu^2+x^2), -0.1);
vi = wH-lambda*Omega*ROTOR;
T = (0.5*BLADES*rho*ASLOPE*CHORD*ROTOR*(Omega*ROTOR)^2*(lambda/2+Theta0*(1/3+Mu^2/2)+ ...
    +THETT*(1/4+Mu^2/4)+Mu/4*(pH/Omega*cos(beta_w)+qH/Omega*sin(beta_w))));
CT = T/(rho*A*(Omega*ROTOR)^2);
V75 = sqrt(vi^2+(0.75*(Omega*ROTOR))^2);
Re = rho*CHORD75*V75/dyn_viscosity;
delta = 0.1166*Re^(-0.2)+0.3/ASLOPE^2*(6*CT/sigma/(1+3/2*Mu^2))^2;

%% forces and moments in the hub-wind frame

H_w = BLADES/2*rho*ASLOPE*CHORD*ROTOR*(Omega*ROTOR)^2*(delta*Mu/(2*ASLOPE)-1/4*Theta0*(2*lambda*Mu+ ...
      +2/3*(pH/Omega*cos(beta_w)+qH/Omega*sin(beta_w)))-THETT/4*(Mu*lambda+1/2*(pH/Omega*cos(beta_w)+ ...
      +qH/Omega*sin(beta_w)))+1/4*(-2*a0/3*(-pH/Omega*sin(beta_w)+qH/Omega*cos(beta_w))+ ...
      -2*lambda*(pH/Omega*cos(beta_w)+qH/Omega*sin(beta_w)))+Mu/4*a0^2);
Y_w = BLADES/2*rho*ASLOPE*CHORD*ROTOR*(Omega*ROTOR)^2*(-1/4*Theta0*(3*a0*Mu+ ...
      -2/3*(-pH/Omega*sin(beta_w)+qH/Omega*cos(beta_w)))-THETT/4*(2*a0*Mu+ ...
      -1/2*(-pH/Omega*sin(beta_w)+qH/Omega*cos(beta_w)))-1/4*(2*a0/3*(pH/Omega*cos(beta_w)+ ...
      +qH/Omega*sin(beta_w))-2*lambda*(-pH/Omega*sin(beta_w)+qH/Omega*cos(beta_w)))-Mu/4*6*a0*lambda);
L_w = 0;
M_w = 0;
Q = k_ind*BLADES/2*rho*ASLOPE*CHORD*ROTOR^2*(Omega*ROTOR)^2*(delta/k_ind/(4*ASLOPE)*(1+Mu^2)-Theta0*(lambda/3+ ...
    +Mu/6*(pH/Omega*cos(beta_w)+qH/Omega*sin(beta_w)))-THETT*lambda/4-1/2*lambda^2+ ...
    +Mu/3*a0*(-pH/Omega*sin(beta_w)+qH/Omega*cos(beta_w))-1/8*(-pH/Omega*sin(beta_w)+ ...
    +qH/Omega*cos(beta_w))^2-1/8*(pH/Omega*cos(beta_w)+qH/Omega*sin(beta_w))^2);


%% back rotation from hub_wind frame to hub-frame

H_H = H_w*cos(beta_w)+Y_w*sin(beta_w);
Y_H = -H_w*sin(beta_w)+Y_w*cos(beta_w);
L_H = L_w*cos(beta_w)-M_w*sin(beta_w);
M_H = L_w*sin(beta_w)+M_w*cos(beta_w);

%% back rotation from hub-frame to body-frame

X = -H_H;
Y = chi*Y_H;
Z = -T;
Frotor = [X Y Z]';
Mrotor = [chi*L_H M_H chi*Q]'+cross(lever_arm_H,Frotor);

== matlab function multi_rotor_sim/MULTIROTOR MODEL/ROTORS FORCE AND MOMENT/ROTOR3/ELECTRICAL EFFICIENCY MODEL ==
  data: Q input; Pe output; Omega input; p00 input; p10 input; p01 input; p20 input; p11 input; p02 input
function Pe = fcn(Q,Omega,p00,p10,p01,p20,p11,p02)
eta_e = p00 + p10*Omega + p01*Q + p20*Omega^2 + p02*Q^2 + p11*Omega*Q;
Psh = Omega*Q;
Pe = Psh/eta_e;

== matlab function multi_rotor_sim/MULTIROTOR MODEL/ROTORS FORCE AND MOMENT/ROTOR3/MATLAB Function ==
  data: BLADES input; Mrotor output; ASLOPE input; CHORD input; CHORD75 input; ROTOR input; a0 input; Theta0 input; THETT input; dyn_viscosity input; k_ind input; STACG input; BLCG input; WLCG input; STAH input; BLH input; WLH input; chi input; rho input; TAS input; omega_TAS input; Frotor output; Q output; omega input; Omega input
function [Mrotor,Frotor,Q] = fcn(BLADES,ASLOPE,CHORD,CHORD75,ROTOR,a0,Theta0,THETT,dyn_viscosity,k_ind,STACG,BLCG,WLCG,STAH,BLH,WLH,chi,rho,TAS,omega_TAS,omega,Omega)

%% preliminary calculations
A = pi*ROTOR^2; % area of rotor disc 
sigma = BLADES*CHORD/(pi*ROTOR); % solidity of rotor 
lever_arm_H = [STACG-STAH BLH-BLCG WLCG-WLH]'; % vector from cg to rotor hub
TAS_H = [1 chi 1]'.*(TAS + cross(omega_TAS,lever_arm_H)); % wind speed at rotor
uH = TAS_H(1);
vH = TAS_H(2);
wH = TAS_H(3);
beta_w = atan2(vH,uH); % sideslip angle 
Mu = sqrt(uH^2+vH^2)/(Omega*ROTOR); % advance ratio
p = omega(1); % roll rate
q = omega(2); % pitch rate
pH = chi*p;
qH = q;

%% thrust calculation

lambda = fzero(@(x) x-wH/(Omega*ROTOR)+0.5*((0.5*BLADES*rho*ASLOPE*CHORD*ROTOR*(Omega*ROTOR)^2*(x/2+ ...
         +Theta0*(1/3+Mu^2/2)+THETT*(1/4+Mu^2/4)+Mu/4*(pH/Omega*cos(beta_w)+ ...
         +qH/Omega*sin(beta_w))))/(rho*A*(Omega*ROTOR)^2))/sqrt(Mu^2+x^2), -0.1);
vi = wH-lambda*Omega*ROTOR;
T = (0.5*BLADES*rho*ASLOPE*CHORD*ROTOR*(Omega*ROTOR)^2*(lambda/2+Theta0*(1/3+Mu^2/2)+ ...
    +THETT*(1/4+Mu^2/4)+Mu/4*(pH/Omega*cos(beta_w)+qH/Omega*sin(beta_w))));
CT = T/(rho*A*(Omega*ROTOR)^2);
V75 = sqrt(vi^2+(0.75*(Omega*ROTOR))^2);
Re = rho*CHORD75*V75/dyn_viscosity;
delta = 0.1166*Re^(-0.2)+0.3/ASLOPE^2*(6*CT/sigma/(1+3/2*Mu^2))^2;

%% forces and moments in the hub-wind frame

H_w = BLADES/2*rho*ASLOPE*CHORD*ROTOR*(Omega*ROTOR)^2*(delta*Mu/(2*ASLOPE)-1/4*Theta0*(2*lambda*Mu+ ...
      +2/3*(pH/Omega*cos(beta_w)+qH/Omega*sin(beta_w)))-THETT/4*(Mu*lambda+1/2*(pH/Omega*cos(beta_w)+ ...
      +qH/Omega*sin(beta_w)))+1/4*(-2*a0/3*(-pH/Omega*sin(beta_w)+qH/Omega*cos(beta_w))+ ...
      -2*lambda*(pH/Omega*cos(beta_w)+qH/Omega*sin(beta_w)))+Mu/4*a0^2);
Y_w = BLADES/2*rho*ASLOPE*CHORD*ROTOR*(Omega*ROTOR)^2*(-1/4*Theta0*(3*a0*Mu+ ...
      -2/3*(-pH/Omega*sin(beta_w)+qH/Omega*cos(beta_w)))-THETT/4*(2*a0*Mu+ ...
      -1/2*(-pH/Omega*sin(beta_w)+qH/Omega*cos(beta_w)))-1/4*(2*a0/3*(pH/Omega*cos(beta_w)+ ...
      +qH/Omega*sin(beta_w))-2*lambda*(-pH/Omega*sin(beta_w)+qH/Omega*cos(beta_w)))-Mu/4*6*a0*lambda);
L_w = 0;
M_w = 0;
Q = k_ind*BLADES/2*rho*ASLOPE*CHORD*ROTOR^2*(Omega*ROTOR)^2*(delta/k_ind/(4*ASLOPE)*(1+Mu^2)-Theta0*(lambda/3+ ...
    +Mu/6*(pH/Omega*cos(beta_w)+qH/Omega*sin(beta_w)))-THETT*lambda/4-1/2*lambda^2+ ...
    +Mu/3*a0*(-pH/Omega*sin(beta_w)+qH/Omega*cos(beta_w))-1/8*(-pH/Omega*sin(beta_w)+ ...
    +qH/Omega*cos(beta_w))^2-1/8*(pH/Omega*cos(beta_w)+qH/Omega*sin(beta_w))^2);


%% back rotation from hub_wind frame to hub-frame

H_H = H_w*cos(beta_w)+Y_w*sin(beta_w);
Y_H = -H_w*sin(beta_w)+Y_w*cos(beta_w);
L_H = L_w*cos(beta_w)-M_w*sin(beta_w);
M_H = L_w*sin(beta_w)+M_w*cos(beta_w);

%% back rotation from hub-frame to body-frame

X = -H_H;
Y = chi*Y_H;
Z = -T;
Frotor = [X Y Z]';
Mrotor = [chi*L_H M_H chi*Q]'+cross(lever_arm_H,Frotor);

== matlab function multi_rotor_sim/MULTIROTOR MODEL/ROTORS FORCE AND MOMENT/ROTOR4/ELECTRICAL EFFICIENCY MODEL ==
  data: Q input; Pe output; Omega input; p00 input; p10 input; p01 input; p20 input; p11 input; p02 input
function Pe = fcn(Q,Omega,p00,p10,p01,p20,p11,p02)
eta_e = p00 + p10*Omega + p01*Q + p20*Omega^2 + p02*Q^2 + p11*Omega*Q;
Psh = Omega*Q;
Pe = Psh/eta_e;

== matlab function multi_rotor_sim/MULTIROTOR MODEL/ROTORS FORCE AND MOMENT/ROTOR4/MATLAB Function ==
  data: BLADES input; Mrotor output; ASLOPE input; CHORD input; CHORD75 input; ROTOR input; a0 input; Theta0 input; THETT input; dyn_viscosity input; k_ind input; STACG input; BLCG input; WLCG input; STAH input; BLH input; WLH input; chi input; rho input; TAS input; omega_TAS input; Frotor output; Q output; omega input; Omega input
function [Mrotor,Frotor,Q] = fcn(BLADES,ASLOPE,CHORD,CHORD75,ROTOR,a0,Theta0,THETT,dyn_viscosity,k_ind,STACG,BLCG,WLCG,STAH,BLH,WLH,chi,rho,TAS,omega_TAS,omega,Omega)

%% preliminary calculations
A = pi*ROTOR^2; % area of rotor disc 
sigma = BLADES*CHORD/(pi*ROTOR); % solidity of rotor 
lever_arm_H = [STACG-STAH BLH-BLCG WLCG-WLH]'; % vector from cg to rotor hub
TAS_H = [1 chi 1]'.*(TAS + cross(omega_TAS,lever_arm_H)); % wind speed at rotor
uH = TAS_H(1);
vH = TAS_H(2);
wH = TAS_H(3);
beta_w = atan2(vH,uH); % sideslip angle 
Mu = sqrt(uH^2+vH^2)/(Omega*ROTOR); % advance ratio
p = omega(1); % roll rate
q = omega(2); % pitch rate
pH = chi*p;
qH = q;

%% thrust calculation

lambda = fzero(@(x) x-wH/(Omega*ROTOR)+0.5*((0.5*BLADES*rho*ASLOPE*CHORD*ROTOR*(Omega*ROTOR)^2*(x/2+ ...
         +Theta0*(1/3+Mu^2/2)+THETT*(1/4+Mu^2/4)+Mu/4*(pH/Omega*cos(beta_w)+ ...
         +qH/Omega*sin(beta_w))))/(rho*A*(Omega*ROTOR)^2))/sqrt(Mu^2+x^2), -0.1);
vi = wH-lambda*Omega*ROTOR;
T = (0.5*BLADES*rho*ASLOPE*CHORD*ROTOR*(Omega*ROTOR)^2*(lambda/2+Theta0*(1/3+Mu^2/2)+ ...
    +THETT*(1/4+Mu^2/4)+Mu/4*(pH/Omega*cos(beta_w)+qH/Omega*sin(beta_w))));
CT = T/(rho*A*(Omega*ROTOR)^2);
V75 = sqrt(vi^2+(0.75*(Omega*ROTOR))^2);
Re = rho*CHORD75*V75/dyn_viscosity;
delta = 0.1166*Re^(-0.2)+0.3/ASLOPE^2*(6*CT/sigma/(1+3/2*Mu^2))^2;

%% forces and moments in the hub-wind frame

H_w = BLADES/2*rho*ASLOPE*CHORD*ROTOR*(Omega*ROTOR)^2*(delta*Mu/(2*ASLOPE)-1/4*Theta0*(2*lambda*Mu+ ...
      +2/3*(pH/Omega*cos(beta_w)+qH/Omega*sin(beta_w)))-THETT/4*(Mu*lambda+1/2*(pH/Omega*cos(beta_w)+ ...
      +qH/Omega*sin(beta_w)))+1/4*(-2*a0/3*(-pH/Omega*sin(beta_w)+qH/Omega*cos(beta_w))+ ...
      -2*lambda*(pH/Omega*cos(beta_w)+qH/Omega*sin(beta_w)))+Mu/4*a0^2);
Y_w = BLADES/2*rho*ASLOPE*CHORD*ROTOR*(Omega*ROTOR)^2*(-1/4*Theta0*(3*a0*Mu+ ...
      -2/3*(-pH/Omega*sin(beta_w)+qH/Omega*cos(beta_w)))-THETT/4*(2*a0*Mu+ ...
      -1/2*(-pH/Omega*sin(beta_w)+qH/Omega*cos(beta_w)))-1/4*(2*a0/3*(pH/Omega*cos(beta_w)+ ...
      +qH/Omega*sin(beta_w))-2*lambda*(-pH/Omega*sin(beta_w)+qH/Omega*cos(beta_w)))-Mu/4*6*a0*lambda);
L_w = 0;
M_w = 0;
Q = k_ind*BLADES/2*rho*ASLOPE*CHORD*ROTOR^2*(Omega*ROTOR)^2*(delta/k_ind/(4*ASLOPE)*(1+Mu^2)-Theta0*(lambda/3+ ...
    +Mu/6*(pH/Omega*cos(beta_w)+qH/Omega*sin(beta_w)))-THETT*lambda/4-1/2*lambda^2+ ...
    +Mu/3*a0*(-pH/Omega*sin(beta_w)+qH/Omega*cos(beta_w))-1/8*(-pH/Omega*sin(beta_w)+ ...
    +qH/Omega*cos(beta_w))^2-1/8*(pH/Omega*cos(beta_w)+qH/Omega*sin(beta_w))^2);


%% back rotation from hub_wind frame to hub-frame

H_H = H_w*cos(beta_w)+Y_w*sin(beta_w);
Y_H = -H_w*sin(beta_w)+Y_w*cos(beta_w);
L_H = L_w*cos(beta_w)-M_w*sin(beta_w);
M_H = L_w*sin(beta_w)+M_w*cos(beta_w);

%% back rotation from hub-frame to body-frame

X = -H_H;
Y = chi*Y_H;
Z = -T;
Frotor = [X Y Z]';
Mrotor = [chi*L_H M_H chi*Q]'+cross(lever_arm_H,Frotor);

== matlab function multi_rotor_sim/MULTIROTOR MODEL/ROTORS FORCE AND MOMENT/ROTOR5/ELECTRICAL EFFICIENCY MODEL ==
  data: Q input; Pe output; Omega input; p00 input; p10 input; p01 input; p20 input; p11 input; p02 input
function Pe = fcn(Q,Omega,p00,p10,p01,p20,p11,p02)
eta_e = p00 + p10*Omega + p01*Q + p20*Omega^2 + p02*Q^2 + p11*Omega*Q;
Psh = Omega*Q;
Pe = Psh/eta_e;
